simulink model "cart_pend"  (R2019a)
settings: Solver=FixedStepAuto  StartTime=0.0  StopTime=25  FixedStep=0.001  RelTol=1e-3
values from neighbouring files (symbols this model uses):
  h = params.h    [prepare_sim.m]
  X0 = [0; 0; pi/12; 0]    [prepare_sim.m]
undefined symbols (not defined in the file or in its folder): Discrete, params, Time, x0, xf
libraries: ctrlSharedLib x1
settings Model: Creator=Piku  LastModifiedBy=Piku

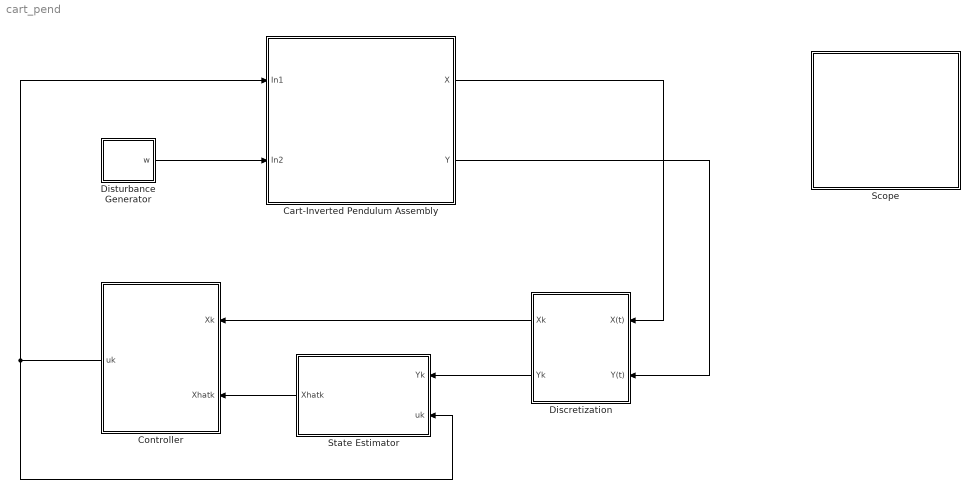
== system cart_pend ==
  Cart-Inverted Pendulum Assembly : Subsystem
      mask Display: image('cart_pendulum.png');
  Controller : Subsystem
  Discretization : Subsystem
  Disturbance Generator : Subsystem
  Scope : Subsystem
  State Estimator : Subsystem
  wires:
  Cart-Inverted Pendulum Assembly/1("X ") -> Discretization/1(X(t))
  Controller/1(uk) -> State Estimator/2(uk), Cart-Inverted Pendulum Assembly/1(In1)
  Cart-Inverted Pendulum Assembly/2(Y) -> Discretization/2(Y(t))
  Discretization/1(Xk) -> Controller/1(" Xk")
  State Estimator/1(Xhatk) -> Controller/2(" Xhatk")
  Disturbance Generator/1(w) -> Cart-Inverted Pendulum Assembly/2(In2)
  Discretization/2(Yk) -> State Estimator/1("Yk ")

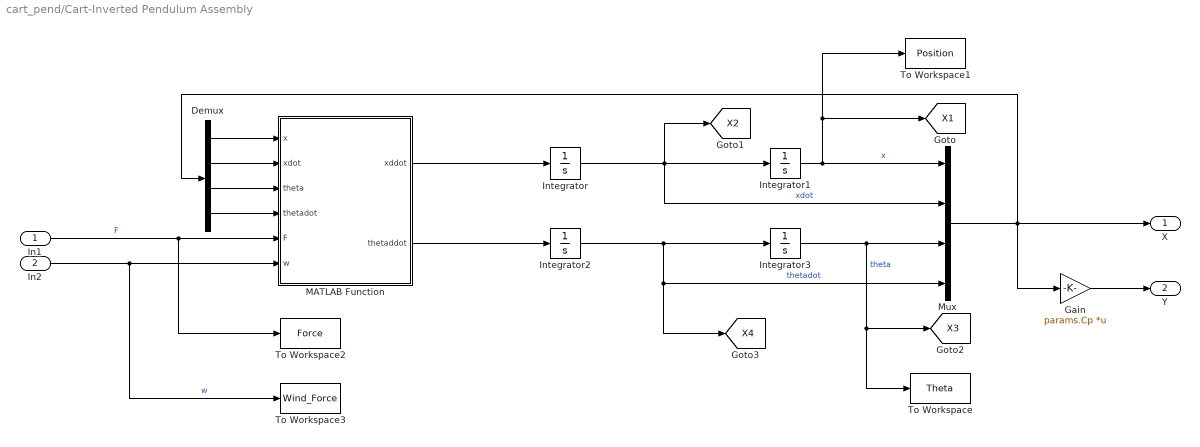
== system cart_pend/Cart-Inverted Pendulum Assembly ==
  In1 : Inport
  In2 : Inport  Port=2  PortDimensions=1
  Demux : Demux
  Gain : Gain  Gain=params.Cp  Multiplication=Matrix(K*u)
  Integrator : Integrator  InitialCondition=X0(2)  LimitOutput=on  UpperSaturationLimit=1e6  LowerSaturationLimit=-1e6
  Integrator1 : Integrator  InitialCondition=X0(1)  UpperSaturationLimit=xf  LowerSaturationLimit=-x0
  Integrator2 : Integrator  InitialCondition=X0(4)  LimitOutput=on  UpperSaturationLimit=1e6  LowerSaturationLimit=-1e6
  Integrator3 : Integrator  InitialCondition=X0(3)  LimitOutput=on  UpperSaturationLimit=pi  LowerSaturationLimit=-pi
  MATLAB Function : MATLAB Function  TreatAsAtomicUnit=on
  Mux : Mux
  To Workspace : ToWorkspace  VariableName=Theta  SaveFormat=Timeseries  SampleTime=-1
  To Workspace1 : ToWorkspace  VariableName=Position  SaveFormat=Timeseries  SampleTime=-1
  To Workspace2 : ToWorkspace  VariableName=Force  SaveFormat=Timeseries  SampleTime=-1
  To Workspace3 : ToWorkspace  VariableName=Wind_Force  SaveFormat=Timeseries  SampleTime=-1
  "X " : Outport  PortDimensions=4
  Y : Outport  Port=2
  tag scope: X1=global, X2=global, X3=global, X4=global
  wires:
  Integrator2/1 -> Integrator3/1, [X4], Mux/4  "thetadot"
  In1/1 -> To Workspace2/1, MATLAB Function/5(F)  "F"
  Integrator3/1 -> Mux/3, To Workspace/1, [X3]  "theta"
  Integrator/1 -> [X2], Mux/2, Integrator1/1  "xdot"
  Integrator1/1 -> [X1], To Workspace1/1, Mux/1  "x"
  Mux/1 -> Gain/1, Demux/1, "X "/1
  MATLAB Function/1(xddot) -> Integrator/1
  MATLAB Function/2(thetaddot) -> Integrator2/1
  Demux/1 -> MATLAB Function/1(x)
  Demux/2 -> MATLAB Function/2(xdot)
  Demux/3 -> MATLAB Function/3(theta)
  Demux/4 -> MATLAB Function/4(thetadot)
  In2/1 -> To Workspace3/1, MATLAB Function/6(w)  "w"
  Gain/1 -> Y/1

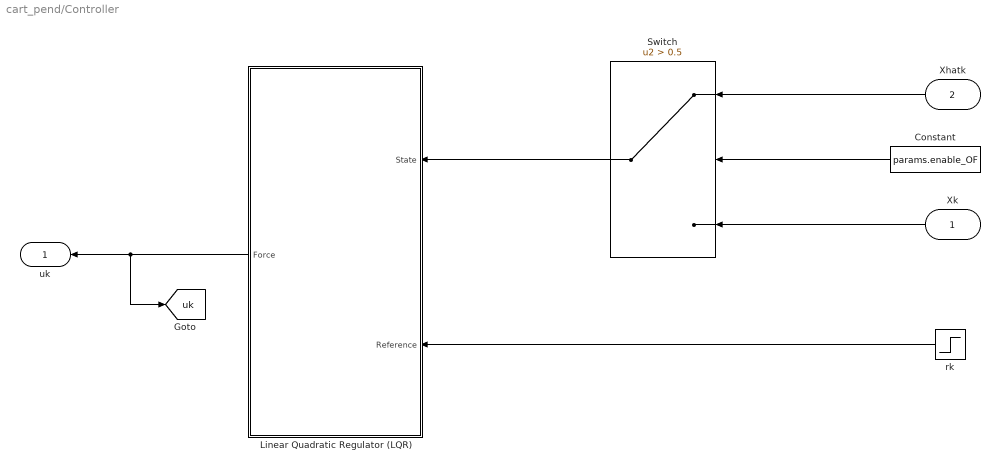
== system cart_pend/Controller ==
  " Xk" : Inport
  " Xhatk" : Inport  Port=2
  Constant : Constant  Value=params.enable_OF
  Linear Quadratic Regulator (LQR) : Subsystem
  Switch : Switch  Criteria=u2 > Threshold  Threshold=0.5
  rk : Step  Time=0  Before=X0(1)  After=10  SampleTime=h
  uk : Outport
  tag scope: uk=global
  wires:
  " Xk"/1 -> Switch/3
  Constant/1 -> Switch/2
  Switch/1 -> Linear Quadratic Regulator (LQR)/1(State)
  " Xhatk"/1 -> Switch/1
  rk/1 -> Linear Quadratic Regulator (LQR)/2("Reference ")
  Linear Quadratic Regulator (LQR)/1(Force) -> [uk], uk/1

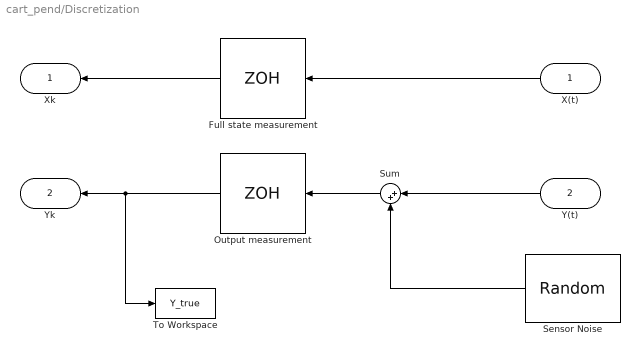
== system cart_pend/Discretization ==
  X(t) : Inport
  Y(t) : Inport  Port=2
  Full state measurement : ZeroOrderHold  SampleTime=h
  Output measurement : ZeroOrderHold  SampleTime=h
  Sensor Noise : UniformRandomNumber  Minimum=-0.005  Maximum=0.005  SampleTime=h
  Sum : Sum  Inputs=|++
  To Workspace : ToWorkspace  VariableName=Y_true  SaveFormat=Timeseries  SampleTime=-1
  Xk : Outport
  Yk : Outport  Port=2
  wires:
  X(t)/1 -> Full state measurement/1
  Full state measurement/1 -> Xk/1
  Output measurement/1 -> To Workspace/1, Yk/1
  Sum/1 -> Output measurement/1
  Y(t)/1 -> Sum/1
  Sensor Noise/1 -> Sum/2

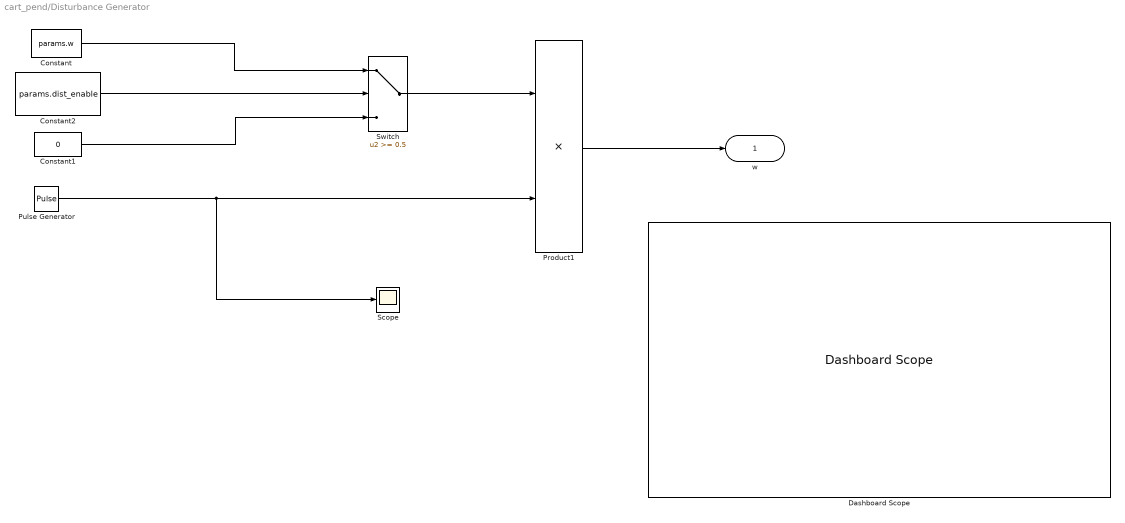
== system cart_pend/Disturbance Generator ==
  Constant : Constant  Value=params.w
  Constant1 : Constant  Value=0
  Constant2 : Constant  Value=params.dist_enable
  Dashboard Scope : DashboardScope  Ymin=0  Ymax=0.02
  Product1 : Product
  Pulse Generator : DiscretePulseGenerator  PulseType=Time based  Period=25  PulseWidth=75  PhaseDelay=10
  Scope : Scope
  Switch : Switch  Threshold=0.5
  w : Outport
  wires:
  Constant2/1 -> Switch/2
  Constant1/1 -> Switch/3
  Constant/1 -> Switch/1
  Switch/1 -> Product1/1
  Product1/1 -> w/1
  Pulse Generator/1 -> Scope/1, Product1/2

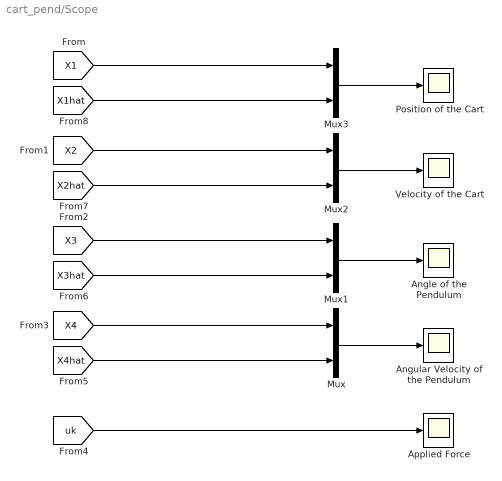
== system cart_pend/Scope ==
  Angle of the Pendulum : Scope
  Angular Velocity of the Pendulum : Scope
  Applied Force : Scope
  Mux{,1..3} (4 alike) : Mux  Inputs=2
  Position of the Cart : Scope
  Velocity of the Cart : Scope
  wires:
  [uk] -> Applied Force/1
  Mux/1 -> Angular Velocity of the Pendulum/1
  [X4] -> Mux/1
  [X4hat] -> Mux/2
  Mux1/1 -> Angle of the Pendulum/1
  [X3] -> Mux1/1
  Mux3/1 -> Position of the Cart/1
  [X1] -> Mux3/1
  [X1hat] -> Mux3/2
  Mux2/1 -> Velocity of the Cart/1
  [X2] -> Mux2/1
  [X2hat] -> Mux2/2
  [X3hat] -> Mux1/2

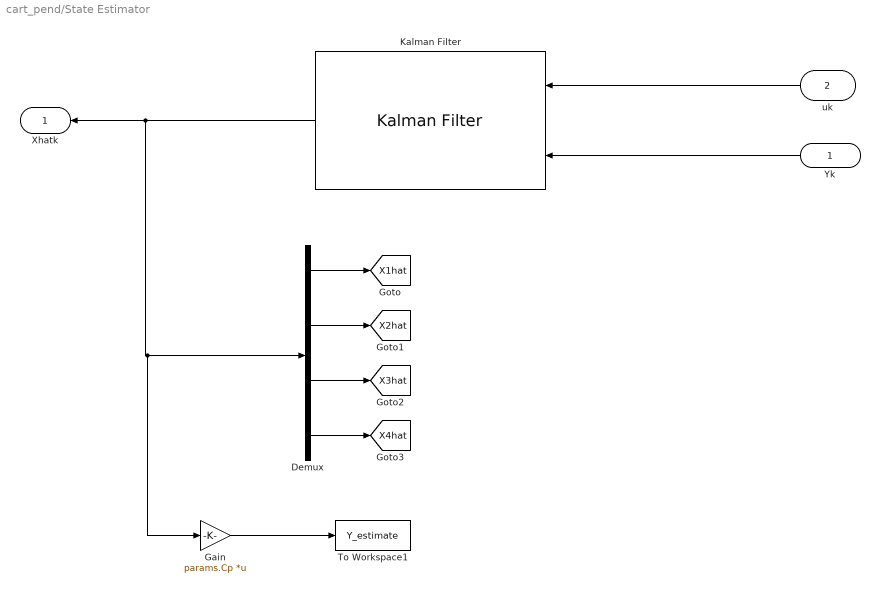
== system cart_pend/State Estimator ==
  "Yk " : Inport  SampleTime=h
  uk : Inport  Port=2  SampleTime=h
  Demux : Demux
  Gain : Gain  Gain=params.Cp  Multiplication=Matrix(K*u)
  "Kalman Filter " : ctrlSharedLib/Kalman Filter  TimeDomain=Discrete-Time  UseCurrentEstimator=on  ModelSource=Individual A, B, C, D matrices  ModelSourceVariable=sysKAL  A=params.AK  B=params.BK  C=params.CK  D=params.DK  NumberOfStates=1  NumberOfInputs=1  NumberOfOutputs=1  InitialEstimateSource=Dialog  X0=X0  P0=10  UseK=off  UseGH=off  NumberOfProcessNoiseInputs=1  G=1  TimeInvariantG=on  H=0  TimeInvariantH=on  Q=params.QK  TimeInvariantQ=on  R=params.RK  TimeInvariantR=on  N=0  TimeInvariantN=on  AddInputPort=on  AddEnablePort=off  OutputEstimatedY=off  OutputP=off  Ts=h
      settings: SourceProductBaseCode=CT
  To Workspace1 : ToWorkspace  VariableName=Y_estimate  SaveFormat=Timeseries  SampleTime=-1
  Xhatk : Outport
  tag scope: X1hat=global, X2hat=global, X3hat=global, X4hat=global
  wires:
  Demux/1 -> [X1hat]
  Demux/2 -> [X2hat]
  Demux/3 -> [X3hat]
  Demux/4 -> [X4hat]
  Gain/1 -> To Workspace1/1
  "Yk "/1 -> "Kalman Filter "/2
  uk/1 -> "Kalman Filter "/1
  "Kalman Filter "/1 -> Gain/1, Demux/1, Xhatk/1

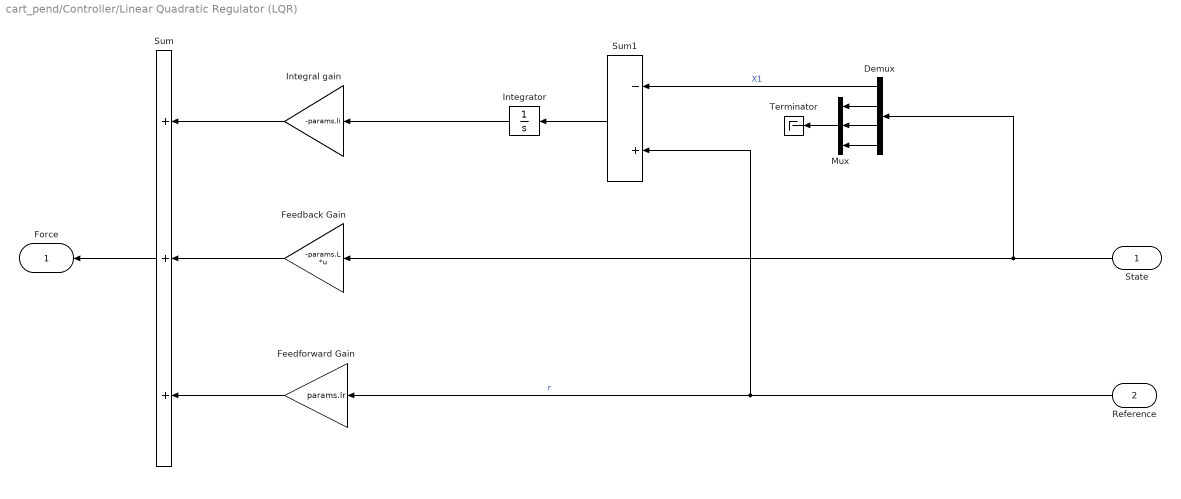
== system cart_pend/Controller/Linear Quadratic Regulator (LQR) ==
  State : Inport
  "Reference " : Inport  Port=2
  Demux : Demux
  Feedback Gain : Gain  Gain=-params.L  Multiplication=Matrix(K*u) (u vector)
  Feedforward Gain : Gain  Gain=params.lr
  Integral gain : Gain  Gain=-params.li
  Integrator : Integrator  InitialCondition=-10  UpperSaturationLimit=1  LowerSaturationLimit=-1
  Mux : Mux  Inputs=3
  Sum : Sum  Inputs=+++
  Sum1 : Sum  Inputs=-+
  Terminator : Terminator
  Force : Outport
  wires:
  Sum/1 -> Force/1
  Demux/1 -> Sum1/1  "X1"
  "Reference "/1 -> Sum1/2, Feedforward Gain/1  "r"
  Feedback Gain/1 -> Sum/2
  State/1 -> Feedback Gain/1, Demux/1
  Sum1/1 -> Integrator/1
  Integrator/1 -> Integral gain/1
  Integral gain/1 -> Sum/1
  Feedforward Gain/1 -> Sum/3
  Demux/4 -> Mux/3
  Mux/1 -> Terminator/1
  Demux/2 -> Mux/1
  Demux/3 -> Mux/2

== matlab function cart_pend/Cart-Inverted Pendulum Assembly/MATLAB Function ==
  data: x input; xddot output; xdot input; theta input; thetadot input; F input; thetaddot output; w input
function [xddot, thetaddot] = fcn(x, xdot, theta, thetadot, F, w)

M   = 0.5;          % Mass of the cart      
m   = 0.2;          % Mass of the inverted pendulum
bc  = 0.1;          % coefficient of friction for cart
l   = 0.3;          % length to the pendulum center of mass
I   = 0.006;        % moment of inertia of the pendulum
bp  = 0.012;        % coefficient of friction for pendulum
g   = 9.8;          % acceleration due to gravity

% Dynamics of the pendulum
ap0 = (I + m*l^2);
ap1 = -(m^2*l^2)/(M+m);
bp0 = (m*l)/(M+m);
bp1 = 0.5*(m^2*l^2)/(M+m);
bp2 = (m*l*bc)/(M+m);
bp3 = bp;
bp4 = -m*g*l; 
bp5 = -l;
thetaddot = (1/(ap0 + ap1*cos(theta)^2))* ( bp0*cos(theta)*(F - w) ...
             - bp1*thetadot^2*sin(2*theta) - bp2*cos(theta)*xdot ...
             - bp3*thetadot - bp4*sin(theta) - bp5*cos(theta)*w );

% Dynamics of the cart
ac0 = M + m;
ac1 = - m^2*l^2/(I + m*l^2);
bc0 = 1;
bc1 = m*l;
bc2 = bc;
bc3 = (bp*m*l)/(I + m*l^2);
bc4 = -0.5*(m^2*l^2*g)/(I + m*l^2);
bc5 = -(m*l^2)/(I + m*l^2);
xddot = (1/(ac0 + ac1*cos(theta)^2))* (bc0*(F - w)...
             - bc1*thetadot^2*sin(theta) - bc2*xdot ...
             - bc3*thetadot*cos(theta) - bc4*sin(2*theta) ...
             - bc5*w*cos(theta)^2 );
end
